simulink model "SimulateBuckConverterModel"  (R2018a)
settings: Solver=ode14x  StartTime=0.0  StopTime=10.0  FixedStep=dt  RelTol=1e-3
values from neighbouring files (symbols this model uses):
  dt = 0.001    [BuckTest.m]    (also in MultiLevelInverterTest_iDesign.m)
  IL_0 = Io*(Vref/Vin)    (= 0.00833333333333)    [BuckTest.m]
  Io = 0.1    [BuckTest.m]
  IoLoaded = 20    [BuckTest.m]
  Kd = 0.00    (= 0)    [BuckTest.m]    (also in MultiLevelInverterTest_iDesign.m)
  Ki = 2.00    (= 2)    [BuckTest.m]    (also in MultiLevelInverterTest_iDesign.m = 0.0002)
  Kp = 0.00    (= 0)    [BuckTest.m]    (also in MultiLevelInverterTest_iDesign.m)
  Vc_0 = Vin    (= 12)    [BuckTest.m]
  Vin = 12    [BuckTest.m]    (also in MultiLevelInverterTest_iDesign.m = 640000)
  Vref = 1    [BuckTest.m]
libraries: simulink x1, Lib_PB_BuckConv_TMATS x1, Lib_Solve_IterNRSolverJC_TMATS x1
settings Model: Creator=tcarsten  LastModifiedBy=mebell
settings SolverCC: AlgebraicLoopSolver=LineSearch
settings CodeAppCC: StateflowObjectComments=on

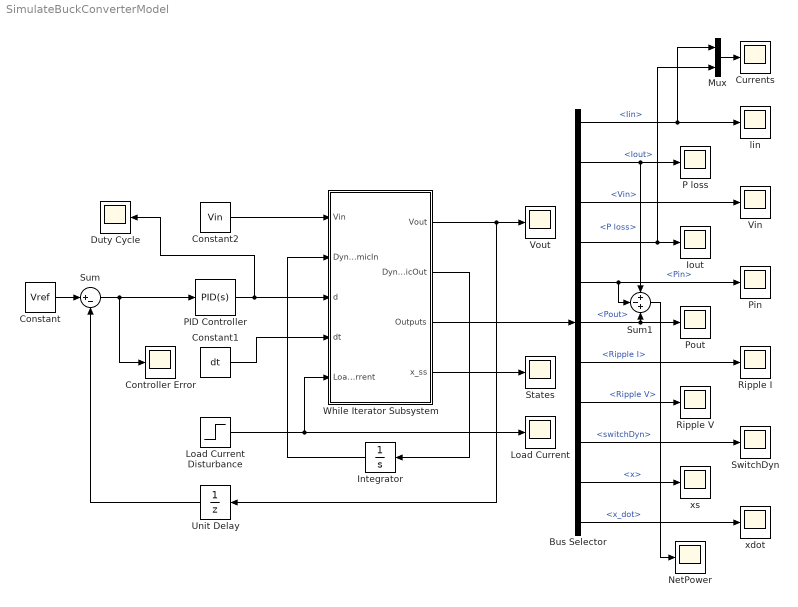
== system SimulateBuckConverterModel ==
  Bus Selector : BusSelector  OutputSignals=Iin,P loss,Vin,Iout,Pin,Pout,Ripple I,Ripple V,switchDyn,x,x_dot
  Constant : Constant  Value=Vref  VectorParams1D=off
  Constant1 : Constant  Value=dt  VectorParams1D=off
  Constant2 : Constant  Value=Vin  VectorParams1D=off
  Controller Error : Scope
  Currents : Scope
  Duty Cycle : Scope
  Integrator : Integrator  InitialCondition=[Vc_0; IL_0]
  Iout : Scope
  Load Current : Scope
  Load Current Disturbance : Step  Time=5  Before=Io  After=IoLoaded  SampleTime=0  VectorParams1D=off
  Mux : Mux  Inputs=2
  NetPower : Scope
  P loss : Scope
  PID Controller : simulink/Continuous/PID Controller  Controller=PID  TimeDomain=Continuous-time  SampleTime=-1  IntegratorMethod=Forward Euler  FilterMethod=Forward Euler  Form=Parallel  UseFilter=on  ControllerParametersSource=internal  P=Kp  I=Ki  D=Kd  N=100  InitialConditionSource=internal  InitialConditionForIntegrator=0  InitialConditionForFilter=0  ExternalReset=none  LimitOutput=on  UpperSaturationLimit=1  LowerSaturationLimit=0  LinearizeAsGain=on  AntiWindupMode=none  Kb=1  TrackingMode=off  Kt=1  PParamMin=[]  PParamMax=[]  IParamMin=[]  IParamMax=[]  DParamMin=[]  DParamMax=[]  NParamMin=[]  NParamMax=[]  KbParamMin=[]  KbParamMax=[]  KtParamMin=[]  KtParamMax=[]  POutMin=[]  POutMax=[]  IOutMin=[]  IOutMax=[]  DOutMin=[]  DOutMax=[]  NOutMin=[]  NOutMax=[]  KbOutMin=[]  KbOutMax=[]  KtOutMin=[]  KtOutMax=[]  IntegratorOutMin=[]  IntegratorOutMax=[]  FilterOutMin=[]  FilterOutMax=[]  SumOutMin=[]  SumOutMax=[]  SumI1OutMin=[]  SumI1OutMax=[]  SumI2OutMin=[]  SumI2OutMax=[]  SumI3OutMin=[]  SumI3OutMax=[]  SumDOutMin=[]  SumDOutMax=[]  SaturationOutMin=[]  SaturationOutMax=[]  IntegratorContinuousStateAttributes=''  IntegratorStateMustResolveToSignalObject=off  IntegratorRTWStateStorageClass=Auto  FilterContinuousStateAttributes=''  FilterStateMustResolveToSignalObject=off  FilterRTWStateStorageClass=Auto  DifferentiatorICPrevScaledInput=0  DifferentiatorOutMin=[]  DifferentiatorOutMax=[]  FilterDiffOutCoefMin=[]  FilterDiffOutCoefMax=[]  SumDenOutMin=[]  SumDenOutMax=[]  SumNumOutMin=[]  SumNumOutMax=[]  ReciprocalOutMin=[]  ReciprocalOutMax=[]  DivideOutMin=[]  DivideOutMax=[]  TunerSelectOption=Transfer Function Based (PID Tuner App)
  Pin : Scope
  Pout : Scope
  Ripple I : Scope
  Ripple V : Scope
  States : Scope
  Sum : Sum  Inputs=|+-
  Sum1 : Sum  Inputs=+-+
  SwitchDyn : Scope
  Unit Delay : UnitDelay  InitialCondition=Vref  SampleTime=-1
  Vin : Scope
  Vout : Scope
  While Iterator Subsystem : Subsystem  TreatAsAtomicUnit=on
  lin : Scope
  xdot : Scope
  xs : Scope
  wires:
  While Iterator Subsystem/2(DynamicOut) -> Integrator/1
  Integrator/1 -> While Iterator Subsystem/2(DynamicIn)
  Constant/1 -> Sum/1
  Sum/1 -> Controller Error/1, PID Controller/1
  PID Controller/1 -> Duty Cycle/1, While Iterator Subsystem/3(d)
  Constant1/1 -> While Iterator Subsystem/4(dt)
  Constant2/1 -> While Iterator Subsystem/1(Vin)
  Load Current Disturbance/1 -> While Iterator Subsystem/5(Load Current), Load Current/1
  Bus Selector/1 -> lin/1, Mux/1  "<Iin>"
  Bus Selector/2 -> Sum1/1, P loss/1  "<P loss>"
  Bus Selector/3 -> Vin/1  "<Vin>"
  Bus Selector/4 -> Mux/2, Iout/1  "<Iout>"
  Bus Selector/5 -> Sum1/2, Pin/1  "<Pin>"
  While Iterator Subsystem/3(Outputs) -> Bus Selector/1
  Bus Selector/6 -> Sum1/3, Pout/1  "<Pout>"
  Bus Selector/7 -> Ripple I/1  "<Ripple I>"
  Bus Selector/8 -> Ripple V/1  "<Ripple V>"
  While Iterator Subsystem/1(Vout) -> Unit Delay/1, Vout/1
  Unit Delay/1 -> Sum/2
  While Iterator Subsystem/4(x_ss) -> States/1
  Bus Selector/9 -> SwitchDyn/1  "<switchDyn>"
  Sum1/1 -> NetPower/1
  Mux/1 -> Currents/1
  Bus Selector/11 -> xdot/1  "<x_dot>"
  Bus Selector/10 -> xs/1  "<x>"

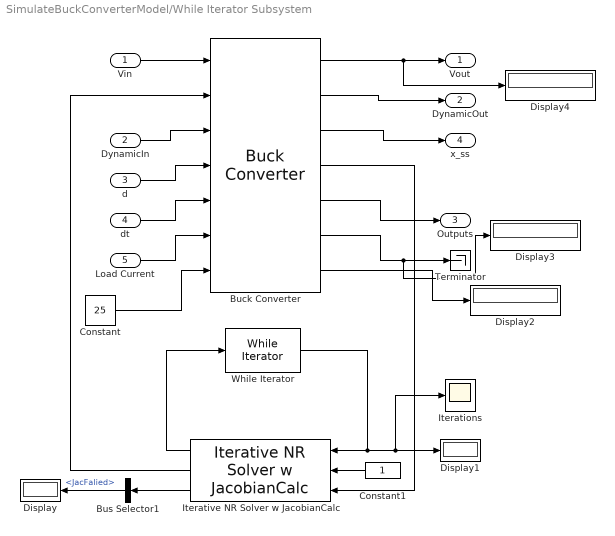
== system SimulateBuckConverterModel/While Iterator Subsystem ==
  Vin : Inport
  DynamicIn : Inport  Port=2
  d : Inport  Port=3
  dt : Inport  Port=4
  Load Current : Inport  Port=5
  Buck Converter : Lib_PB_BuckConv_TMATS/Buck Converter  Pdis_M=1  C_M=600e-6  L_M=0.3e-6  Ron_M=1.5e-3  RC_M=1e-3  RL_M=1e-3  QgTotal_M=2e-9  Vgate_M=0.5  TRise_M=4e-9  TFall_M=6e-9  Fsw_M=1e6  Trr_M=0  TempIn=Celsius
  Bus Selector1 : BusSelector  OutputSignals=JacFalied
  Constant : Constant  Value=25
  Constant1 : Constant
  Display{,1..4} (5 alike) : Display
  Iterations : Scope
  Iterative NR Solver w JacobianCalc : Lib_Solve_IterNRSolverJC_TMATS/Iterative NR Solver w JacobianCalc  SJac_Per_M=[0.01]  SNR_IC_M=IL_0  SNR_DX_M=5  SNR_Mx_M=100000  SNR_Mn_M=0.0001  SJacobianAttempts_M=20  Cond_Limits_M=0.000001
  Terminator : Terminator
  While Iterator : WhileIterator  MaxIters=10000  WhileBlockType=do-while  ShowIterationPort=on
  Vout : Outport
  DynamicOut : Outport  Port=2
  Outputs : Outport  Port=3
  x_ss : Outport  Port=4
  wires:
  Buck Converter/2 -> DynamicOut/1
  dt/1 -> Buck Converter/5
  DynamicIn/1 -> Buck Converter/3
  Buck Converter/6 -> Display3/1, Terminator/1
  Vin/1 -> Buck Converter/1
  d/1 -> Buck Converter/4
  Bus Selector1/1 -> Display/1  "<JacFalied>"
  While Iterator/1 -> Iterative NR Solver w JacobianCalc/1, Iterations/1, Display1/1
  Constant1/1 -> Iterative NR Solver w JacobianCalc/2
  Buck Converter/4 -> Iterative NR Solver w JacobianCalc/3
  Iterative NR Solver w JacobianCalc/1 -> While Iterator/1
  Iterative NR Solver w JacobianCalc/2 -> Buck Converter/2
  Iterative NR Solver w JacobianCalc/3 -> Bus Selector1/1
  Buck Converter/5 -> Outputs/1
  Load Current/1 -> Buck Converter/6
  Buck Converter/3 -> x_ss/1
  Buck Converter/7 -> Display2/1
  Constant/1 -> Buck Converter/7
  Buck Converter/1 -> Display4/1, Vout/1
